simulink model "CraneModel"  (R2020b)
settings: Solver=ode45  StartTime=0.0  StopTime=50  MaxStep=1e-5  RelTol=1e-4
values from neighbouring files (symbols this model uses):
  g = 9.81    [ThongSo.m]    (also in ThongSo_Change.m)
  L = 0.305    [ThongSo.m]    (also in ThongSo_Change.m = 0.8)
  M = 1    [ThongSo.m]    (also in ThongSo_Change.m = 5)
  m = 0.8    [ThongSo.m]    (also in ThongSo_Change.m = 1.5)
  theta0 = 0    [ThongSo.m]    (also in ThongSo_Change.m)
  theta0_dot = 0    [ThongSo.m]    (also in ThongSo_Change.m)
  theta0_dotdot = 0    [ThongSo.m]    (also in ThongSo_Change.m)
  x0 = 0    [ThongSo.m]    (also in ThongSo_Change.m)
  x0_dot = 0    [ThongSo.m]    (also in ThongSo_Change.m)
  x0_dotdot = 0    [ThongSo.m]    (also in ThongSo_Change.m)
undefined symbols (not defined in the file or in its folder): sigbuilder_block
settings Model: Creator=chemi  LastModifiedBy=chemi

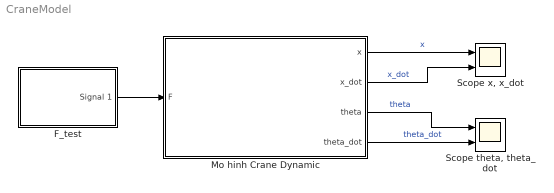
== system CraneModel ==
  F_test : Subsystem  Tag=STV Subsys  LoadFcn=sigbuilder_block('load');  StartFcn=sigbuilder_block('start');  StopFcn=sigbuilder_block('stop');  ClipboardFcn=sigbuilder_block('clipboard');  mask(Sigbuilder block){tuvar=[0:10]}
      mask help: Simulink:masks:SigbuilderBlock_MD
      mask init:
      | if ~strcmp(get_param(bdroot(gcbh),'SimulationStatus'),'stopped') tuvar = sigbuilder_block('maskInit'); end
      settings: CopyFcn=sigbuilder_block('copy');  DeleteFcn=sigbuilder_block('delete');  ModelCloseFcn=sigbuilder_block('modelClose');  PreSaveFcn=sigbuilder_block('preSave');  PauseFcn=sigbuilder_block('pause');  ContinueFcn=sigbuilder_block('continue');  NameChangeFcn=sigbuilder_block('namechange');  OpenFcn=sigbuilder_block('open',[283.5 152.25 550.5 359.25 ]);  CloseFcn=sigbuilder_block('close');
      mask Display: plot(0, 0, 100, 100,[2, 2, 32, 32, 2], [68, 8, 8, 68, 68],[32, 2], [38, 38], [32, 19, 2],[53, 60, 44], [32, 17, 17, 2],[16, 16, 31, 31]);txt = getActiveGroup(gcbh);text(2, 100, txt,'verticalAlignment', 'top');
  Mo hinh Crane Dynamic : Subsystem
  "Scope theta, theta_dot" : Scope  NumInputPorts=2
  "Scope x, x_dot" : Scope  NumInputPorts=2
  wires:
  Mo hinh Crane Dynamic/1(x) -> "Scope x, x_dot"/1  "x"
  Mo hinh Crane Dynamic/2(x_dot) -> "Scope x, x_dot"/2  "x_dot"
  Mo hinh Crane Dynamic/3(theta) -> "Scope theta, theta_dot"/1  "theta"
  Mo hinh Crane Dynamic/4(theta_dot) -> "Scope theta, theta_dot"/2  "theta_dot"
  F_test/1(Signal 1) -> Mo hinh Crane Dynamic/1(F)

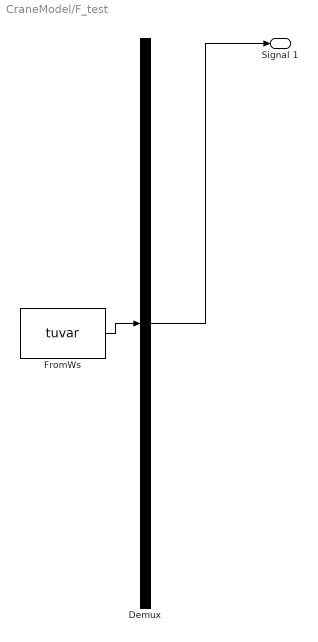
== system CraneModel/F_test ==
  Demux : Demux  Tag=STV Demux  Outputs=1
      settings: DisplayOption=none
  FromWs : FromWorkspace  Tag=STV FromWs  VariableName=tuvar
      SigBuilderData=|
      | common.afterFinalStr = 'Extrapolate'
      | common.sampleTime = 0
      | dataSet.timeRange = [0 50]
      | dataSet.name = 'Group 1'
      | sbobj.Groups.Name = 'Group 1'
      | sbobj.Groups.Signals.Name = 'Signal 1'
      | sbobj.Groups.Signals.XData = [0 8 8 14 14 22 22 30 30 50]
      | sbobj.Groups.Signals.YData = [200 200 -150 -150 130 130 300 300 80 80]
      | sbobj.Groups.TimeRange = [0 50]
  Signal 1 : Outport  Tag=STV Outport  VectorParamsAs1DForOutWhenUnconnected=off
  wires:
  Demux/1 -> Signal 1/1
  FromWs/1 -> Demux/1

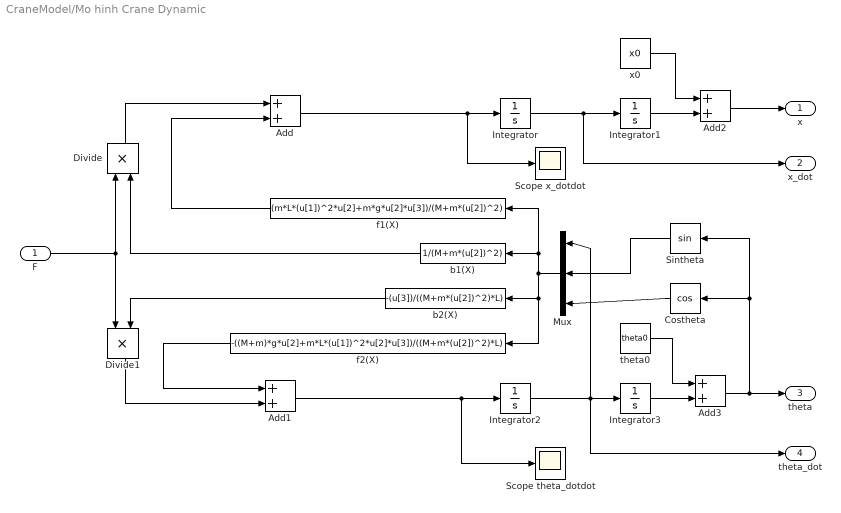
== system CraneModel/Mo hinh Crane Dynamic ==
  F : Inport
  Add{,1..3} (4 alike) : Sum
  Costheta : Trigonometry  Operator=cos
  Divide : Product  Inputs=**
  Divide1 : Product  Inputs=**
  Integrator : Integrator  InitialCondition=x0_dotdot
  Integrator1 : Integrator  InitialCondition=x0_dot
  Integrator2 : Integrator  InitialCondition=theta0_dotdot
  Integrator3 : Integrator  InitialCondition=theta0_dot
  Mux : Mux  Inputs=3
  Scope theta_dotdot : Scope
  Scope x_dotdot : Scope
  Sintheta : Trigonometry
  b1(X) : Fcn  Expr=1/(M+m*(u[2])^2)
  b2(X) : Fcn  Expr=-(u[3])/((M+m*(u[2])^2)*L)
  f1(X) : Fcn  Expr=(m*L*(u[1])^2*u[2]+m*g*u[2]*u[3])/(M+m*(u[2])^2)
  f2(X) : Fcn  Expr=-((M+m)*g*u[2]+m*L*(u[1])^2*u[2]*u[3])/((M+m*(u[2])^2)*L)
  theta0 : Constant  Value=theta0
  x0 : Constant  Value=x0
  x : Outport
  x_dot : Outport  Port=2
  theta : Outport  Port=3
  theta_dot : Outport  Port=4
  wires:
  Integrator1/1 -> Add2/2
  Integrator/1 -> x_dot/1, Integrator1/1
  Integrator2/1 -> theta_dot/1, Mux/1, Integrator3/1
  F/1 -> Divide/1, Divide1/1
  Mux/1 -> f1(X)/1, b1(X)/1, b2(X)/1, f2(X)/1
  Add/1 -> Scope x_dotdot/1, Integrator/1
  b1(X)/1 -> Divide/2
  Add1/1 -> Scope theta_dotdot/1, Integrator2/1
  f2(X)/1 -> Add1/1
  Divide1/1 -> Add1/2
  b2(X)/1 -> Divide1/2
  Divide/1 -> Add/1
  f1(X)/1 -> Add/2
  Add2/1 -> x/1
  x0/1 -> Add2/1
  Integrator3/1 -> Add3/2
  theta0/1 -> Add3/1
  Add3/1 -> Sintheta/1, Costheta/1, theta/1
  Sintheta/1 -> Mux/2
  Costheta/1 -> Mux/3
